simulink model "Y6MultirotorLQGSimulation2"  (R2019b)
settings: Solver=VariableStepAuto  StartTime=0.0  StopTime=500  RelTol=1e-3
values from neighbouring files (symbols this model uses):
  Time = 100    [Simulation.m]
undefined symbols (not defined in the file or in its folder): Cr, DiscIntNeverNeededParam, Discrete, Kdt, Kidt, N, Rv, T
libraries: ctrlSharedLib x1
settings Model: Creator=oscar  LastModifiedBy=alexd
settings SolverCC: AlgebraicLoopSolver=LineSearch
settings DataIOCC: ReturnWorkspaceOutputs=off
settings DebuggingCC: ArithmeticOperatorsInVariantConditions=warning
settings SFSimCC: SimUseLocalCustomCode=off  CustomCodeUndefinedFunction=UseInterfaceOnly
settings RTWCC: RTWUseLocalCustomCode=off

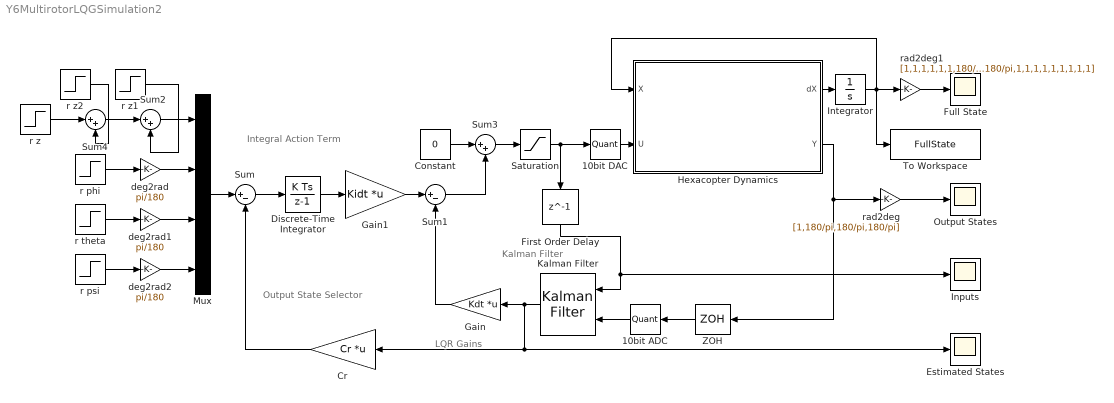
== system Y6MultirotorLQGSimulation2 ==
  note: LQR Gains
  note: Kalman Filter
  note: Integral Action Term
  note: Output State Selector
  10bit ADC : Quantizer  QuantizationInterval=3.3/((2^10)-1)
  10bit DAC : Quantizer  QuantizationInterval=3.3/((2^10)-1)
  Constant : Constant  Value=0
  Cr : Gain  Gain=Cr  Multiplication=Matrix(K*u)
  Discrete-Time Integrator : DiscreteIntegrator  SampleTime=T  ICPrevOutput=DiscIntNeverNeededParam  ICPrevScaledInput=DiscIntNeverNeededParam
  Estimated States : Scope
  First Order Delay : Delay  DelayLength=1  SampleTime=T
  Full State : Scope
  Gain : Gain  Gain=Kdt  Multiplication=Matrix(K*u)
  Gain1 : Gain  Gain=Kidt  Multiplication=Matrix(K*u)
  Hexacopter Dynamics : MATLAB Function  TreatAsAtomicUnit=on
  Inputs : Scope
  Integrator : Integrator  InitialCondition=[0;0;0;0;0;0;0;0;0;0;0;0;0;0;0;0;0;0]
  Kalman Filter : ctrlSharedLib/Kalman Filter  TimeDomain=Discrete-Time  UseCurrentEstimator=on  ModelSource=LTI State-Space Variable  ModelSourceVariable=sysdt  A=0.95  B=1  C=1  D=0  NumberOfStates=1  NumberOfInputs=1  NumberOfOutputs=1  InitialEstimateSource=Dialog  X0=0  P0=10  UseK=off  UseGH=off  NumberOfProcessNoiseInputs=1  G=1  TimeInvariantG=on  H=0  TimeInvariantH=on  Q=Rw  TimeInvariantQ=on  R=Rv  TimeInvariantR=on  N=N  TimeInvariantN=on  AddInputPort=on  AddEnablePort=off  OutputEstimatedY=off  OutputP=off  Ts=-1
      settings: SourceProductBaseCode=CT
  Mux : Mux
  Output States : Scope
  Saturation : Saturate  UpperLimit=1000  LowerLimit=0
  Sum : Sum  Inputs=|+-
  Sum1 : Sum  Inputs=|+-
  Sum2 : Sum  Inputs=|++
  Sum3 : Sum  Inputs=|++
  Sum4 : Sum  Inputs=|++
  To Workspace : ToWorkspace  VariableName=FullState  SaveFormat=Timeseries  SampleTime=-1
  ZOH : ZeroOrderHold  SampleTime=T
  deg2rad : Gain  Gain=pi/180  SaturateOnIntegerOverflow=on  OutDataTypeStr=Inherit: Same as input  ParamDataTypeStr=Inherit: Same as input
  deg2rad1 : Gain  Gain=pi/180  SaturateOnIntegerOverflow=on  OutDataTypeStr=Inherit: Same as input  ParamDataTypeStr=Inherit: Same as input
  deg2rad2 : Gain  Gain=pi/180  SaturateOnIntegerOverflow=on  OutDataTypeStr=Inherit: Same as input  ParamDataTypeStr=Inherit: Same as input
  r phi : Step  Time=200  After=5  SampleTime=0
  r psi : Step  Time=0  After=0  SampleTime=0
  r theta : Step  Time=0  After=0  SampleTime=0
  r z : Step  Time=50  After=2  SampleTime=0
  r z1 : Step  Time=150  After=-2  SampleTime=0
  r z2 : Step  Time=100  After=2  SampleTime=0
  rad2deg : Gain  Gain=[1,180/pi,180/pi,180/pi]  SaturateOnIntegerOverflow=on  OutDataTypeStr=Inherit: Same as input  ParamDataTypeStr=Inherit: Same as input
  rad2deg1 : Gain  Gain=[1,1,1,1,1,1,180/pi,180/pi,180/pi,1,1,1,1,1,1,1,1,1]  SaturateOnIntegerOverflow=on  OutDataTypeStr=Inherit: Same as input  ParamDataTypeStr=Inherit: Same as input
  wires:
  Hexacopter Dynamics/1(dX) -> Integrator/1
  Integrator/1 -> rad2deg1/1, Hexacopter Dynamics/1(X), To Workspace/1
  Kalman Filter/1 -> Gain/1, Cr/1, Estimated States/1
  Gain/1 -> Sum1/2
  Gain1/1 -> Sum1/1
  Hexacopter Dynamics/2(Y) -> rad2deg/1, ZOH/1
  Constant/1 -> Sum3/1
  r phi/1 -> deg2rad/1
  deg2rad/1 -> Mux/2
  r theta/1 -> deg2rad1/1
  r psi/1 -> deg2rad2/1
  deg2rad2/1 -> Mux/4
  deg2rad1/1 -> Mux/3
  rad2deg/1 -> Output States/1
  rad2deg1/1 -> Full State/1
  Sum3/1 -> Saturation/1
  Sum/1 -> Discrete-Time Integrator/1
  Discrete-Time Integrator/1 -> Gain1/1
  Cr/1 -> Sum/2
  Sum1/1 -> Sum3/2
  Saturation/1 -> 10bit DAC/1, First Order Delay/1
  ZOH/1 -> 10bit ADC/1
  Mux/1 -> Sum/1
  10bit DAC/1 -> Hexacopter Dynamics/2(U)
  10bit ADC/1 -> Kalman Filter/2
  First Order Delay/1 -> Inputs/1, Kalman Filter/1
  Sum2/1 -> Mux/1
  r z1/1 -> Sum2/2
  r z/1 -> Sum4/1
  r z2/1 -> Sum4/2
  Sum4/1 -> Sum2/1

== matlab function Y6MultirotorLQGSimulation2/Hexacopter Dynamics ==
  data: dX output; X input; U input; Y output
function [dX,Y]  = Hexacopter_Dynamics(X,U)
%% Mass of the Multirotor in Kilograms as taken from the CAD

M = 2100/1000; 
g = 9.81;

%% Dimensions of Multirotor

L1 = 22/100; % along X-axis Distance from left and right motor pair to center of mass
L2 = 15/100; % along Y-axis Vertical Distance from left and right motor pair to center of mass
L3 = 30/100; % along Y-axis Distance from motor pair to center of mass

%%  Mass Moment of Inertia as Taken from the CAD

Ixx = 3.094E+05;
Ixy = 45.147;
Ixz = 2.309;
Iyx = 45.147;
Iyy = 4.204E+05;
Iyz = 832.833;
Izx = 2.309;
Izy = 832.833;
Izz = 1.464E+05;

%% Inertia Matrix and Diagolalisation CAD model coordinate system rotated 90 degrees about X

I = [Izx Izy Izz;
     Ixx Ixy Ixz;
     Iyx Iyy Iyz];
 
Idiag = diag(I)/10000;
 
Ixx = Idiag(1);
Iyy = Idiag(2);
Izz = Idiag(3);

%% Motor Thrust and Torque Constants (To be determined experimentally)

Kw = 0.85;
Ktau =  2.46*(10^-12);
Kthrust =  3.7155*(10^-7);
Kthrust2 = -3.7327*(10^-4);
Mtau = (1/44.22);
Ku = 515.5;


%% Air resistance damping coeeficients

Dxx = 0.02;
Dyy = 0.02;
Dzz = 0.1;

%% X = [x xdot y ydot z zdot phi phidot theta thetadot psi psidot w1 w2 w3 w4 w5 w6]

x = X(1);
xdot = X(2);
y = X(3);
ydot = X(4);
z = X(5);
zdot = X(6);

phi = X(7); 
theta = X(8);
psi = X(9);

p = X(10);
q = X(11);
r = X(12);

w1 = X(13);
w2 = X(14);
w3 = X(15);
w4 = X(16);
w5 = X(17);
w6 = X(18);

%% Initialise Outputs

dX = zeros(18,1);
Y = zeros(4,1);

%% Motor Dynamics: dX = [w1dot w2dot w3dot w4dot w5dot w6dot], U = Duty Cycle of the pwm signal 0-100%

dX(13) = -(1/Mtau)*w1 + Ku*U(1);
dX(14) = -(1/Mtau)*w2 + Ku*U(2);
dX(15) = -(1/Mtau)*w3 + Ku*U(3);
dX(16) = -(1/Mtau)*w4 + Ku*U(4);
dX(17) = -(1/Mtau)*w5 + Ku*U(5);
dX(18) = -(1/Mtau)*w6 + Ku*U(6);

%% Motor Forces and Torques

F = zeros(6,1);
T = zeros(6,1);

F(1)= Kw*Kthrust*(w1^2) + Kthrust2*w1;
F(2)= Kthrust*(w2^2) + Kthrust2*w2;
F(3)= Kw*Kthrust*(w3^2)+ Kthrust2*w3;
F(4)= Kthrust*(w4^2) + Kthrust2*w4;
F(5)= Kw*Kthrust*(w5^2) + Kthrust2*w5;
F(6)= Kthrust*(w6^2) + Kthrust2*w6;

T(1)= Ktau*(w1^2);
T(2)= -Ktau*(w2^2);
T(3)= -Ktau*(w3^2);
T(4)= Ktau*(w4^2);
T(5)= Ktau*(w5^2);
T(6)= -Ktau*(w6^2);

Fn = sum(F);
Tn = sum(T);

%% First Order Direvatives dX = [xdot ydot zdot phidot thetadot psidot]

dX(1) = X(2);
dX(3) = X(4);
dX(5) = X(6);
dX(7) = p + q*(sin(phi)*tan(theta)) + r*(cos(phi)*tan(theta));
dX(8) = q*cos(phi) - r*sin(phi);
dX(9) = q*(sin(phi)/cos(theta)) + r*(cos(phi)/cos(theta));

%% Second Order Direvatives: dX = [xddot yddot zddot pdot qdot rdot]

dX(2) = Fn/M*(cos(phi)*sin(theta)*cos(psi)) + Fn/M*(sin(phi)*sin(psi)) - (Dxx/M)*xdot;
dX(4) = Fn/M*(cos(phi)*sin(theta)*sin(psi)) - Fn/M*(sin(phi)*cos(psi)) - (Dyy/M)*ydot;
dX(6) = Fn/M*(cos(phi)*cos(theta)) - g - (Dzz/M)*zdot;

dX(10) = (L1/Ixx)*((F(1)+F(2)) - (F(3)+F(4))) - ((Izz-Iyy)/Ixx)*(r*q); 
dX(11) = (L3/Iyy)*(F(5)+F(6)) - (L2/Iyy)*(F(1)+F(2)+F(3)+F(4)) - ((Izz-Ixx)/Iyy)*(p*r);
dX(12) = Tn/Izz - ((Iyy-Ixx)/Izz)*(p*q);

%% Measured States

Y(1) = z;
Y(2) = phi;
Y(3) = theta;
Y(4) = psi;

end
